simulink model "Y_Model_2_Loads"  (R2018b)
settings: Solver=VariableStepAuto  StartTime=0.0  StopTime=sim_t  RelTol=1e-3
values from neighbouring files (symbols this model uses):
  dt = 5e-5    (= 5e-05)    [Y_multi_sim_loads.m]
  L = ones(num_sims, num_loads) * L_max    [Y_multi_sim_loads.m]
  P = rand(num_sims, num_loads) * (P_max - P_min) + P_min    [Y_multi_sim_loads.m]
  R = ones(num_sims, num_loads) * R_max    [Y_multi_sim_loads.m]
libraries: powerlib x65, powerlib_meascontrol x13
settings Model: Creator=mitchell  LastModifiedBy=mitchell

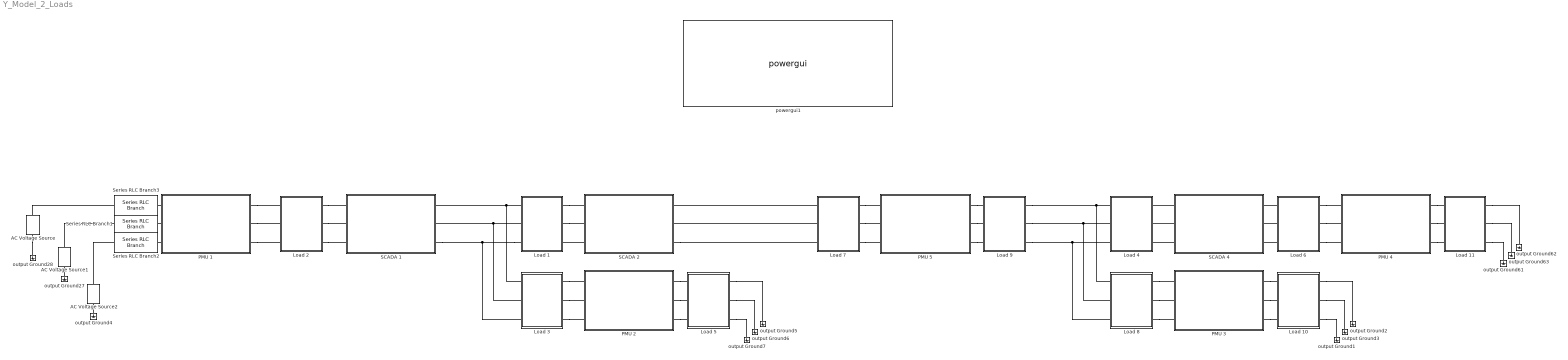
== system Y_Model_2_Loads ==
  AC Voltage Source : powerlib/Electrical Sources/AC Voltage Source  Amplitude=240  Phase=0  Frequency=50  SampleTime=0  Measurements=None  BusType=swing  Pref=10e3  Qref=0  Qmin=-inf  Qmax=+inf
  AC Voltage Source1 : powerlib/Electrical Sources/AC Voltage Source  Amplitude=240  Phase=-120  Frequency=50  SampleTime=0  Measurements=None  BusType=swing  Pref=10e3  Qref=0  Qmin=-inf  Qmax=+inf
  AC Voltage Source2 : powerlib/Electrical Sources/AC Voltage Source  Amplitude=240  Phase=-240  Frequency=50  SampleTime=0  Measurements=None  BusType=swing  Pref=10e3  Qref=0  Qmin=-inf  Qmax=+inf
  Load 1 : Subsystem
  Load 10 : Subsystem
  Load 11 : Subsystem
  Load 2 : Subsystem
  Load 3 : Subsystem
  Load 4 : Subsystem
  Load 5 : Subsystem
  Load 6 : Subsystem
  Load 7 : Subsystem
  Load 8 : Subsystem
  Load 9 : Subsystem
  PMU 1 : Subsystem
  PMU 2 : Subsystem
  PMU 3 : Subsystem
  PMU 4 : Subsystem
  PMU 5 : Subsystem
  SCADA 1 : Subsystem
  SCADA 2 : Subsystem
  SCADA 4 : Subsystem
  Series RLC Branch1 : powerlib/Elements/Series RLC Branch  LConnTagsString=__new0  RConnTagsString=__new0  BranchType=R  Resistance=1  Inductance=L(4)  SetiL0=off  InitialCurrent=0  Capacitance=0  Setx0=off  InitialVoltage=0  Measurements=None
  Series RLC Branch2 : powerlib/Elements/Series RLC Branch  LConnTagsString=__new0  RConnTagsString=__new0  BranchType=R  Resistance=1  Inductance=L(4)  SetiL0=off  InitialCurrent=0  Capacitance=0  Setx0=off  InitialVoltage=0  Measurements=None
  Series RLC Branch3 : powerlib/Elements/Series RLC Branch  LConnTagsString=__new0  RConnTagsString=__new0  BranchType=R  Resistance=1  Inductance=L(4)  SetiL0=off  InitialCurrent=0  Capacitance=0  Setx0=off  InitialVoltage=0  Measurements=None
  output Ground{1..7,27..28,61..63} (12 alike) : powerlib/Elements/Ground  LConnTagsString=a
      settings: SourceProductName=Simscape Electrical
  powergui1 : powerlib/powergui  Priority=1  SimulationMode=Discrete  SampleTime=dt  frequency=60  Iterations=500  frequencyindice=50  Pbase=100e6  ErrMax=0.0001  UnitsV=kV  UnitsW=MW  buscounter=1  FunctionMessages=off  echomessages=off  EnableUseOfTLC=off  CurrentSourceSwitches=off  DisableSnubberDevices=off  DisableRonSwitches=off  DisableVfSwitches=off  DisplayEquations=off  SolverType=Tustin/Backward Euler (TBE)  Interpol=off  ExternalGateDelay=off  methode=off  Ts=100  x0status=blocks  SPID=on  SwTol=0  HookPort=off  RestoreLinks=warning  ResistiveCurrentMeasurement=off  Frange=[0:2:500]  Ylog=off  Xlog=on  ShowGrid=off  save=off  variable=ZData  structure=0  ZoomFFT=off  StartTime=0.0  cycles=1  DisplayStyle=1  fundamental=60  FreqAxis=off  MaxFrequency=1000  frequencyindicesteady=1  RmsSteady=1  display=off
  connections:
  output Ground4/LConn1 -- AC Voltage Source2/LConn1
  output Ground27/LConn1 -- AC Voltage Source1/LConn1
  AC Voltage Source/LConn1 -- output Ground28/LConn1
  Series RLC Branch1/RConn1 -- PMU 1/LConn2
  Series RLC Branch2/RConn1 -- PMU 1/LConn3
  Load 3/LConn2 -- SCADA 1/RConn2 -- Load 1/LConn2
  Load 1/RConn1 -- SCADA 2/LConn1
  SCADA 2/LConn3 -- Load 1/RConn3
  AC Voltage Source2/RConn1 -- Series RLC Branch2/LConn1
  Series RLC Branch1/LConn1 -- AC Voltage Source1/RConn1
  Series RLC Branch3/LConn1 -- AC Voltage Source/RConn1
  PMU 1/LConn1 -- Series RLC Branch3/RConn1
  Load 1/LConn1 -- SCADA 1/RConn1 -- Load 3/LConn1
  PMU 1/RConn3 -- Load 2/LConn3
  PMU 1/RConn2 -- Load 2/LConn2
  PMU 1/RConn1 -- Load 2/LConn1
  Load 1/LConn3 -- SCADA 1/RConn3 -- Load 3/LConn3
  Load 2/RConn1 -- SCADA 1/LConn1
  Load 2/RConn2 -- SCADA 1/LConn2
  Load 2/RConn3 -- SCADA 1/LConn3
  Load 3/RConn1 -- PMU 2/LConn1
  Load 3/RConn2 -- PMU 2/LConn2
  Load 3/RConn3 -- PMU 2/LConn3
  PMU 2/RConn3 -- Load 5/LConn3
  PMU 2/RConn2 -- Load 5/LConn2
  PMU 2/RConn1 -- Load 5/LConn1
  Load 7/LConn2 -- SCADA 2/RConn2
  Load 7/LConn1 -- SCADA 2/RConn1
  SCADA 2/RConn3 -- Load 7/LConn3
  Load 7/RConn3 -- PMU 5/LConn3
  Load 7/RConn1 -- PMU 5/LConn1
  PMU 5/RConn2 -- Load 9/LConn2
  PMU 5/RConn1 -- Load 9/LConn1
  Load 7/RConn2 -- PMU 5/LConn2
  PMU 5/RConn3 -- Load 9/LConn3
  Load 1/RConn2 -- SCADA 2/LConn2
  Load 5/RConn2 -- output Ground6/LConn1
  Load 5/RConn1 -- output Ground5/LConn1
  Load 5/RConn3 -- output Ground7/LConn1
  Load 8/LConn2 -- Load 9/RConn2 -- Load 4/LConn2
  Load 4/LConn3 -- Load 9/RConn3 -- Load 8/LConn3
  Load 8/LConn1 -- Load 9/RConn1 -- Load 4/LConn1
  SCADA 4/LConn1 -- Load 4/RConn1
  Load 10/RConn3 -- output Ground1/LConn1
  Load 10/RConn2 -- output Ground3/LConn1
  SCADA 4/LConn3 -- Load 4/RConn3
  Load 10/RConn1 -- output Ground2/LConn1
  PMU 3/RConn2 -- Load 10/LConn2
  PMU 3/RConn3 -- Load 10/LConn3
  SCADA 4/LConn2 -- Load 4/RConn2
  Load 8/RConn1 -- PMU 3/LConn1
  PMU 3/RConn1 -- Load 10/LConn1
  Load 8/RConn2 -- PMU 3/LConn2
  Load 8/RConn3 -- PMU 3/LConn3
  Load 11/RConn2 -- output Ground63/LConn1
  Load 6/RConn1 -- PMU 4/LConn1
  PMU 4/RConn2 -- Load 11/LConn2
  Load 11/RConn3 -- output Ground61/LConn1
  PMU 4/RConn1 -- Load 11/LConn1
  Load 11/RConn1 -- output Ground62/LConn1
  PMU 4/RConn3 -- Load 11/LConn3
  Load 6/RConn2 -- PMU 4/LConn2
  Load 6/RConn3 -- PMU 4/LConn3
  Load 6/LConn1 -- SCADA 4/RConn1
  Load 6/LConn2 -- SCADA 4/RConn2
  Load 6/LConn3 -- SCADA 4/RConn3

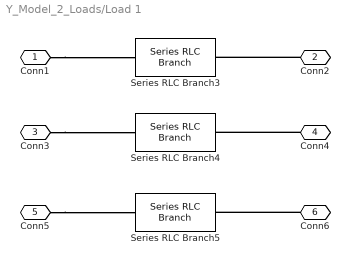
== system Y_Model_2_Loads/Load 1 ==
  Series RLC Branch3 : powerlib/Elements/Series RLC Branch  LConnTagsString=__new0  RConnTagsString=__new0  BranchType=RL  Resistance=R(1)  Inductance=L(1)  SetiL0=off  InitialCurrent=0  Capacitance=0  Setx0=off  InitialVoltage=0  Measurements=None
  Series RLC Branch4 : powerlib/Elements/Series RLC Branch  LConnTagsString=__new0  RConnTagsString=__new0  BranchType=RL  Resistance=R(1)  Inductance=L(1)  SetiL0=off  InitialCurrent=0  Capacitance=0  Setx0=off  InitialVoltage=0  Measurements=None
  Series RLC Branch5 : powerlib/Elements/Series RLC Branch  LConnTagsString=__new0  RConnTagsString=__new0  BranchType=RL  Resistance=R(1)  Inductance=L(1)  SetiL0=off  InitialCurrent=0  Capacitance=0  Setx0=off  InitialVoltage=0  Measurements=None
  Conn1 : PMIOPort  Side=Left
  Conn2 : PMIOPort  Port=2  Side=Right
  Conn3 : PMIOPort  Port=3  Side=Left
  Conn4 : PMIOPort  Port=4  Side=Right
  Conn5 : PMIOPort  Port=5  Side=Left
  Conn6 : PMIOPort  Port=6  Side=Right
  connections:
  Conn5/RConn1 -- Series RLC Branch5/LConn1
  Conn4/RConn1 -- Series RLC Branch4/RConn1
  Conn2/RConn1 -- Series RLC Branch3/RConn1
  Conn3/RConn1 -- Series RLC Branch4/LConn1
  Conn6/RConn1 -- Series RLC Branch5/RConn1
  Conn1/RConn1 -- Series RLC Branch3/LConn1

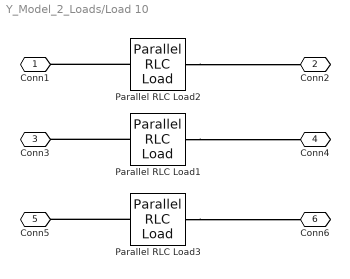
== system Y_Model_2_Loads/Load 10 ==
  Parallel RLC Load1 : powerlib/Elements/Parallel RLC Load  LConnTagsString=a  RConnTagsString=__new0  NominalVoltage=240  NominalFrequency=60  ActivePower=P(10)  InductivePower=P(10)/10  CapacitivePower=0  Setx0=off  InitialVoltage=0  SetiL0=off  InitialCurrent=0  Measurements=None  LoadType=constant Z
      settings: AttributesFormatString=\n  SourceProductName=Simscape Power Systems  SourceProductBaseCode=PS
  Parallel RLC Load2 : powerlib/Elements/Parallel RLC Load  LConnTagsString=a  RConnTagsString=__new0  NominalVoltage=240  NominalFrequency=60  ActivePower=P(10)  InductivePower=P(10)/10  CapacitivePower=0  Setx0=off  InitialVoltage=0  SetiL0=off  InitialCurrent=0  Measurements=None  LoadType=constant Z
      settings: AttributesFormatString=\n  SourceProductName=Simscape Power Systems  SourceProductBaseCode=PS
  Parallel RLC Load3 : powerlib/Elements/Parallel RLC Load  LConnTagsString=a  RConnTagsString=__new0  NominalVoltage=240  NominalFrequency=60  ActivePower=P(10)  InductivePower=P(10)/10  CapacitivePower=0  Setx0=off  InitialVoltage=0  SetiL0=off  InitialCurrent=0  Measurements=None  LoadType=constant Z
      settings: AttributesFormatString=\n  SourceProductName=Simscape Power Systems  SourceProductBaseCode=PS
  Conn1 : PMIOPort  Side=Left
  Conn2 : PMIOPort  Port=2  Side=Right
  Conn3 : PMIOPort  Port=3  Side=Left
  Conn4 : PMIOPort  Port=4  Side=Right
  Conn5 : PMIOPort  Port=5  Side=Left
  Conn6 : PMIOPort  Port=6  Side=Right
  connections:
  Parallel RLC Load3/LConn1 -- Conn5/RConn1
  Parallel RLC Load1/LConn1 -- Conn3/RConn1
  Parallel RLC Load2/LConn1 -- Conn1/RConn1
  Parallel RLC Load2/RConn1 -- Conn2/RConn1
  Parallel RLC Load1/RConn1 -- Conn4/RConn1
  Parallel RLC Load3/RConn1 -- Conn6/RConn1

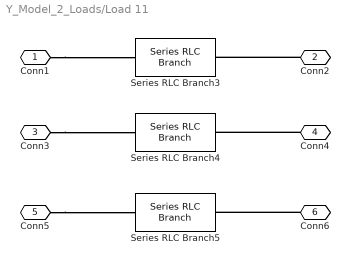
== system Y_Model_2_Loads/Load 11 ==
  Series RLC Branch3 : powerlib/Elements/Series RLC Branch  LConnTagsString=__new0  RConnTagsString=__new0  BranchType=RL  Resistance=R(4)  Inductance=L(4)  SetiL0=off  InitialCurrent=0  Capacitance=0  Setx0=off  InitialVoltage=0  Measurements=None
  Series RLC Branch4 : powerlib/Elements/Series RLC Branch  LConnTagsString=__new0  RConnTagsString=__new0  BranchType=RL  Resistance=R(4)  Inductance=L(4)  SetiL0=off  InitialCurrent=0  Capacitance=0  Setx0=off  InitialVoltage=0  Measurements=None
  Series RLC Branch5 : powerlib/Elements/Series RLC Branch  LConnTagsString=__new0  RConnTagsString=__new0  BranchType=RL  Resistance=R(4)  Inductance=L(4)  SetiL0=off  InitialCurrent=0  Capacitance=0  Setx0=off  InitialVoltage=0  Measurements=None
  Conn1 : PMIOPort  Side=Left
  Conn2 : PMIOPort  Port=2  Side=Right
  Conn3 : PMIOPort  Port=3  Side=Left
  Conn4 : PMIOPort  Port=4  Side=Right
  Conn5 : PMIOPort  Port=5  Side=Left
  Conn6 : PMIOPort  Port=6  Side=Right
  connections:
  Conn5/RConn1 -- Series RLC Branch5/LConn1
  Conn4/RConn1 -- Series RLC Branch4/RConn1
  Conn2/RConn1 -- Series RLC Branch3/RConn1
  Conn3/RConn1 -- Series RLC Branch4/LConn1
  Conn6/RConn1 -- Series RLC Branch5/RConn1
  Conn1/RConn1 -- Series RLC Branch3/LConn1

== system Y_Model_2_Loads/Load 2 ==
  Series RLC Branch3 : powerlib/Elements/Series RLC Branch  LConnTagsString=__new0  RConnTagsString=__new0  BranchType=RL  Resistance=R(2)  Inductance=L(2)  SetiL0=off  InitialCurrent=0  Capacitance=0  Setx0=off  InitialVoltage=0  Measurements=None
  Series RLC Branch4 : powerlib/Elements/Series RLC Branch  LConnTagsString=__new0  RConnTagsString=__new0  BranchType=RL  Resistance=R(2)  Inductance=L(2)  SetiL0=off  InitialCurrent=0  Capacitance=0  Setx0=off  InitialVoltage=0  Measurements=None
  Series RLC Branch5 : powerlib/Elements/Series RLC Branch  LConnTagsString=__new0  RConnTagsString=__new0  BranchType=RL  Resistance=R(2)  Inductance=L(2)  SetiL0=off  InitialCurrent=0  Capacitance=0  Setx0=off  InitialVoltage=0  Measurements=None
  Conn1 : PMIOPort  Side=Left
  Conn2 : PMIOPort  Port=2  Side=Right
  Conn3 : PMIOPort  Port=3  Side=Left
  Conn4 : PMIOPort  Port=4  Side=Right
  Conn5 : PMIOPort  Port=5  Side=Left
  Conn6 : PMIOPort  Port=6  Side=Right
  connections:
  Conn5/RConn1 -- Series RLC Branch5/LConn1
  Conn4/RConn1 -- Series RLC Branch4/RConn1
  Conn2/RConn1 -- Series RLC Branch3/RConn1
  Conn3/RConn1 -- Series RLC Branch4/LConn1
  Conn6/RConn1 -- Series RLC Branch5/RConn1
  Conn1/RConn1 -- Series RLC Branch3/LConn1

== system Y_Model_2_Loads/Load 3 ==
  Series RLC Branch3 : powerlib/Elements/Series RLC Branch  LConnTagsString=__new0  RConnTagsString=__new0  BranchType=RL  Resistance=R(3)  Inductance=L(3)  SetiL0=off  InitialCurrent=0  Capacitance=0  Setx0=off  InitialVoltage=0  Measurements=None
  Series RLC Branch4 : powerlib/Elements/Series RLC Branch  LConnTagsString=__new0  RConnTagsString=__new0  BranchType=RL  Resistance=R(3)  Inductance=L(3)  SetiL0=off  InitialCurrent=0  Capacitance=0  Setx0=off  InitialVoltage=0  Measurements=None
  Series RLC Branch5 : powerlib/Elements/Series RLC Branch  LConnTagsString=__new0  RConnTagsString=__new0  BranchType=RL  Resistance=R(3)  Inductance=L(3)  SetiL0=off  InitialCurrent=0  Capacitance=0  Setx0=off  InitialVoltage=0  Measurements=None
  Conn1 : PMIOPort  Side=Left
  Conn2 : PMIOPort  Port=2  Side=Right
  Conn3 : PMIOPort  Port=3  Side=Left
  Conn4 : PMIOPort  Port=4  Side=Right
  Conn5 : PMIOPort  Port=5  Side=Left
  Conn6 : PMIOPort  Port=6  Side=Right
  connections:
  Conn5/RConn1 -- Series RLC Branch5/LConn1
  Conn4/RConn1 -- Series RLC Branch4/RConn1
  Conn2/RConn1 -- Series RLC Branch3/RConn1
  Conn3/RConn1 -- Series RLC Branch4/LConn1
  Conn6/RConn1 -- Series RLC Branch5/RConn1
  Conn1/RConn1 -- Series RLC Branch3/LConn1

== system Y_Model_2_Loads/Load 4 ==
  Series RLC Branch3 : powerlib/Elements/Series RLC Branch  LConnTagsString=__new0  RConnTagsString=__new0  BranchType=RL  Resistance=R(1)  Inductance=L(1)  SetiL0=off  InitialCurrent=0  Capacitance=0  Setx0=off  InitialVoltage=0  Measurements=None
  Series RLC Branch4 : powerlib/Elements/Series RLC Branch  LConnTagsString=__new0  RConnTagsString=__new0  BranchType=RL  Resistance=R(1)  Inductance=L(1)  SetiL0=off  InitialCurrent=0  Capacitance=0  Setx0=off  InitialVoltage=0  Measurements=None
  Series RLC Branch5 : powerlib/Elements/Series RLC Branch  LConnTagsString=__new0  RConnTagsString=__new0  BranchType=RL  Resistance=R(1)  Inductance=L(1)  SetiL0=off  InitialCurrent=0  Capacitance=0  Setx0=off  InitialVoltage=0  Measurements=None
  Conn1 : PMIOPort  Side=Left
  Conn2 : PMIOPort  Port=2  Side=Right
  Conn3 : PMIOPort  Port=3  Side=Left
  Conn4 : PMIOPort  Port=4  Side=Right
  Conn5 : PMIOPort  Port=5  Side=Left
  Conn6 : PMIOPort  Port=6  Side=Right
  connections:
  Conn5/RConn1 -- Series RLC Branch5/LConn1
  Conn4/RConn1 -- Series RLC Branch4/RConn1
  Conn2/RConn1 -- Series RLC Branch3/RConn1
  Conn3/RConn1 -- Series RLC Branch4/LConn1
  Conn6/RConn1 -- Series RLC Branch5/RConn1
  Conn1/RConn1 -- Series RLC Branch3/LConn1

== system Y_Model_2_Loads/Load 5 ==
  Parallel RLC Load1 : powerlib/Elements/Parallel RLC Load  LConnTagsString=a  RConnTagsString=__new0  NominalVoltage=240  NominalFrequency=60  ActivePower=P(5)  InductivePower=P(5)/10  CapacitivePower=0  Setx0=off  InitialVoltage=0  SetiL0=off  InitialCurrent=0  Measurements=None  LoadType=constant Z
      settings: AttributesFormatString=\n  SourceProductName=Simscape Power Systems  SourceProductBaseCode=PS
  Parallel RLC Load2 : powerlib/Elements/Parallel RLC Load  LConnTagsString=a  RConnTagsString=__new0  NominalVoltage=240  NominalFrequency=60  ActivePower=P(5)  InductivePower=P(5)/10  CapacitivePower=0  Setx0=off  InitialVoltage=0  SetiL0=off  InitialCurrent=0  Measurements=None  LoadType=constant Z
      settings: AttributesFormatString=\n  SourceProductName=Simscape Power Systems  SourceProductBaseCode=PS
  Parallel RLC Load3 : powerlib/Elements/Parallel RLC Load  LConnTagsString=a  RConnTagsString=__new0  NominalVoltage=240  NominalFrequency=60  ActivePower=P(5)  InductivePower=P(5)/10  CapacitivePower=0  Setx0=off  InitialVoltage=0  SetiL0=off  InitialCurrent=0  Measurements=None  LoadType=constant Z
      settings: AttributesFormatString=\n  SourceProductName=Simscape Power Systems  SourceProductBaseCode=PS
  Conn1 : PMIOPort  Side=Left
  Conn2 : PMIOPort  Port=2  Side=Right
  Conn3 : PMIOPort  Port=3  Side=Left
  Conn4 : PMIOPort  Port=4  Side=Right
  Conn5 : PMIOPort  Port=5  Side=Left
  Conn6 : PMIOPort  Port=6  Side=Right
  connections:
  Parallel RLC Load2/LConn1 -- Conn5/RConn1
  Conn4/RConn1 -- Parallel RLC Load1/RConn1
  Parallel RLC Load3/RConn1 -- Conn2/RConn1
  Parallel RLC Load1/LConn1 -- Conn3/RConn1
  Conn6/RConn1 -- Parallel RLC Load2/RConn1
  Parallel RLC Load3/LConn1 -- Conn1/RConn1

== system Y_Model_2_Loads/Load 6 ==
  Series RLC Branch3 : powerlib/Elements/Series RLC Branch  LConnTagsString=__new0  RConnTagsString=__new0  BranchType=RL  Resistance=R(3)  Inductance=L(3)  SetiL0=off  InitialCurrent=0  Capacitance=0  Setx0=off  InitialVoltage=0  Measurements=None
  Series RLC Branch4 : powerlib/Elements/Series RLC Branch  LConnTagsString=__new0  RConnTagsString=__new0  BranchType=RL  Resistance=R(3)  Inductance=L(3)  SetiL0=off  InitialCurrent=0  Capacitance=0  Setx0=off  InitialVoltage=0  Measurements=None
  Series RLC Branch5 : powerlib/Elements/Series RLC Branch  LConnTagsString=__new0  RConnTagsString=__new0  BranchType=RL  Resistance=R(3)  Inductance=L(3)  SetiL0=off  InitialCurrent=0  Capacitance=0  Setx0=off  InitialVoltage=0  Measurements=None
  Conn1 : PMIOPort  Side=Left
  Conn2 : PMIOPort  Port=2  Side=Right
  Conn3 : PMIOPort  Port=3  Side=Left
  Conn4 : PMIOPort  Port=4  Side=Right
  Conn5 : PMIOPort  Port=5  Side=Left
  Conn6 : PMIOPort  Port=6  Side=Right
  connections:
  Conn5/RConn1 -- Series RLC Branch5/LConn1
  Conn4/RConn1 -- Series RLC Branch4/RConn1
  Conn2/RConn1 -- Series RLC Branch3/RConn1
  Conn3/RConn1 -- Series RLC Branch4/LConn1
  Conn6/RConn1 -- Series RLC Branch5/RConn1
  Conn1/RConn1 -- Series RLC Branch3/LConn1

== system Y_Model_2_Loads/Load 7 ==
  Series RLC Branch3 : powerlib/Elements/Series RLC Branch  LConnTagsString=__new0  RConnTagsString=__new0  BranchType=RL  Resistance=R(3)  Inductance=L(3)  SetiL0=off  InitialCurrent=0  Capacitance=0  Setx0=off  InitialVoltage=0  Measurements=None
  Series RLC Branch4 : powerlib/Elements/Series RLC Branch  LConnTagsString=__new0  RConnTagsString=__new0  BranchType=RL  Resistance=R(3)  Inductance=L(3)  SetiL0=off  InitialCurrent=0  Capacitance=0  Setx0=off  InitialVoltage=0  Measurements=None
  Series RLC Branch5 : powerlib/Elements/Series RLC Branch  LConnTagsString=__new0  RConnTagsString=__new0  BranchType=RL  Resistance=R(3)  Inductance=L(3)  SetiL0=off  InitialCurrent=0  Capacitance=0  Setx0=off  InitialVoltage=0  Measurements=None
  Conn1 : PMIOPort  Side=Left
  Conn2 : PMIOPort  Port=2  Side=Right
  Conn3 : PMIOPort  Port=3  Side=Left
  Conn4 : PMIOPort  Port=4  Side=Right
  Conn5 : PMIOPort  Port=5  Side=Left
  Conn6 : PMIOPort  Port=6  Side=Right
  connections:
  Conn5/RConn1 -- Series RLC Branch5/LConn1
  Conn4/RConn1 -- Series RLC Branch4/RConn1
  Conn2/RConn1 -- Series RLC Branch3/RConn1
  Conn3/RConn1 -- Series RLC Branch4/LConn1
  Conn6/RConn1 -- Series RLC Branch5/RConn1
  Conn1/RConn1 -- Series RLC Branch3/LConn1

== system Y_Model_2_Loads/Load 8 ==
  Series RLC Branch3 : powerlib/Elements/Series RLC Branch  LConnTagsString=__new0  RConnTagsString=__new0  BranchType=RL  Resistance=R(3)  Inductance=L(3)  SetiL0=off  InitialCurrent=0  Capacitance=0  Setx0=off  InitialVoltage=0  Measurements=None
  Series RLC Branch4 : powerlib/Elements/Series RLC Branch  LConnTagsString=__new0  RConnTagsString=__new0  BranchType=RL  Resistance=R(3)  Inductance=L(3)  SetiL0=off  InitialCurrent=0  Capacitance=0  Setx0=off  InitialVoltage=0  Measurements=None
  Series RLC Branch5 : powerlib/Elements/Series RLC Branch  LConnTagsString=__new0  RConnTagsString=__new0  BranchType=RL  Resistance=R(3)  Inductance=L(3)  SetiL0=off  InitialCurrent=0  Capacitance=0  Setx0=off  InitialVoltage=0  Measurements=None
  Conn1 : PMIOPort  Side=Left
  Conn2 : PMIOPort  Port=2  Side=Right
  Conn3 : PMIOPort  Port=3  Side=Left
  Conn4 : PMIOPort  Port=4  Side=Right
  Conn5 : PMIOPort  Port=5  Side=Left
  Conn6 : PMIOPort  Port=6  Side=Right
  connections:
  Conn5/RConn1 -- Series RLC Branch5/LConn1
  Conn4/RConn1 -- Series RLC Branch4/RConn1
  Conn2/RConn1 -- Series RLC Branch3/RConn1
  Conn3/RConn1 -- Series RLC Branch4/LConn1
  Conn6/RConn1 -- Series RLC Branch5/RConn1
  Conn1/RConn1 -- Series RLC Branch3/LConn1

== system Y_Model_2_Loads/Load 9 ==
  Series RLC Branch3 : powerlib/Elements/Series RLC Branch  LConnTagsString=__new0  RConnTagsString=__new0  BranchType=RL  Resistance=R(4)  Inductance=L(4)  SetiL0=off  InitialCurrent=0  Capacitance=0  Setx0=off  InitialVoltage=0  Measurements=None
  Series RLC Branch4 : powerlib/Elements/Series RLC Branch  LConnTagsString=__new0  RConnTagsString=__new0  BranchType=RL  Resistance=R(4)  Inductance=L(4)  SetiL0=off  InitialCurrent=0  Capacitance=0  Setx0=off  InitialVoltage=0  Measurements=None
  Series RLC Branch5 : powerlib/Elements/Series RLC Branch  LConnTagsString=__new0  RConnTagsString=__new0  BranchType=RL  Resistance=R(4)  Inductance=L(4)  SetiL0=off  InitialCurrent=0  Capacitance=0  Setx0=off  InitialVoltage=0  Measurements=None
  Conn1 : PMIOPort  Side=Left
  Conn2 : PMIOPort  Port=2  Side=Right
  Conn3 : PMIOPort  Port=3  Side=Left
  Conn4 : PMIOPort  Port=4  Side=Right
  Conn5 : PMIOPort  Port=5  Side=Left
  Conn6 : PMIOPort  Port=6  Side=Right
  connections:
  Conn5/RConn1 -- Series RLC Branch5/LConn1
  Conn4/RConn1 -- Series RLC Branch4/RConn1
  Conn2/RConn1 -- Series RLC Branch3/RConn1
  Conn3/RConn1 -- Series RLC Branch4/LConn1
  Conn6/RConn1 -- Series RLC Branch5/RConn1
  Conn1/RConn1 -- Series RLC Branch3/LConn1

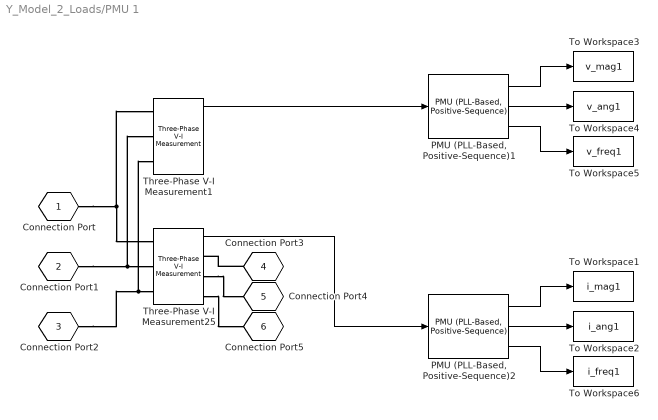
== system Y_Model_2_Loads/PMU 1 ==
  "PMU (PLL-Based, Positive-Sequence)1" : powerlib_meascontrol/Measurements/PMU (PLL-Based, Positive-Sequence)  nominalFrequency=50  samplingRate=64  reportingFactor=64
      settings: SourceProductName=Simscape Electrical  SourceProductBaseCode=PS
  "PMU (PLL-Based, Positive-Sequence)2" : powerlib_meascontrol/Measurements/PMU (PLL-Based, Positive-Sequence)  nominalFrequency=50  samplingRate=64  reportingFactor=64
      settings: SourceProductName=Simscape Electrical  SourceProductBaseCode=PS
  Three-Phase V-I Measurement1 : powerlib/Measurements/Three-Phase V-I Measurement  VoltageMeasurement=phase-to-ground  SetLabelV=off  LabelV=Vabc  Vpu=off  VpuLL=off  CurrentMeasurement=no  SetLabelI=off  LabelI=Iabc  Ipu=off  Pbase=100e6  Vbase=500e3  OutputType=Complex  PhasorSimulation=off  PSBequivalent=0
      settings: SourceProductName=Simscape Electrical
  Three-Phase V-I Measurement25 : powerlib/Measurements/Three-Phase V-I Measurement  VoltageMeasurement=no  SetLabelV=off  LabelV=Vabc  Vpu=off  VpuLL=off  CurrentMeasurement=yes  SetLabelI=off  LabelI=Iabc  Ipu=off  Pbase=100e6  Vbase=500e3  OutputType=Complex  PhasorSimulation=off  PSBequivalent=0
      settings: SourceProductName=Simscape Electrical
  To Workspace1 : ToWorkspace  VariableName=i_mag1  SampleTime=-1
  To Workspace2 : ToWorkspace  VariableName=i_ang1  SampleTime=-1
  To Workspace3 : ToWorkspace  VariableName=v_mag1  SampleTime=-1
  To Workspace4 : ToWorkspace  VariableName=v_ang1  SampleTime=-1
  To Workspace5 : ToWorkspace  VariableName=v_freq1  SampleTime=-1
  To Workspace6 : ToWorkspace  VariableName=i_freq1  SampleTime=-1
  Connection Port : PMIOPort  Tag=PMCPort  Side=Left
  Connection Port1 : PMIOPort  Tag=PMCPort  Port=2  Side=Left
  Connection Port2 : PMIOPort  Tag=PMCPort  Port=3  Side=Left
  Connection Port3 : PMIOPort  Tag=PMCPort  Port=4  Side=Right
  Connection Port4 : PMIOPort  Tag=PMCPort  Port=5  Side=Right
  Connection Port5 : PMIOPort  Tag=PMCPort  Port=6  Side=Right
  wires:
  "PMU (PLL-Based, Positive-Sequence)1"/3 -> To Workspace5/1
  "PMU (PLL-Based, Positive-Sequence)1"/2 -> To Workspace4/1
  "PMU (PLL-Based, Positive-Sequence)1"/1 -> To Workspace3/1
  "PMU (PLL-Based, Positive-Sequence)2"/3 -> To Workspace6/1
  "PMU (PLL-Based, Positive-Sequence)2"/1 -> To Workspace1/1
  "PMU (PLL-Based, Positive-Sequence)2"/2 -> To Workspace2/1
  Three-Phase V-I Measurement25/1 -> "PMU (PLL-Based, Positive-Sequence)2"/1
  Three-Phase V-I Measurement1/1 -> "PMU (PLL-Based, Positive-Sequence)1"/1
  connections:
  Connection Port/RConn1 -- Three-Phase V-I Measurement1/LConn1 -- Three-Phase V-I Measurement25/LConn1
  Connection Port1/RConn1 -- Three-Phase V-I Measurement25/LConn2 -- Three-Phase V-I Measurement1/LConn2
  Connection Port2/RConn1 -- Three-Phase V-I Measurement1/LConn3 -- Three-Phase V-I Measurement25/LConn3
  Connection Port3/RConn1 -- Three-Phase V-I Measurement25/RConn1
  Three-Phase V-I Measurement25/RConn2 -- Connection Port4/RConn1
  Three-Phase V-I Measurement25/RConn3 -- Connection Port5/RConn1

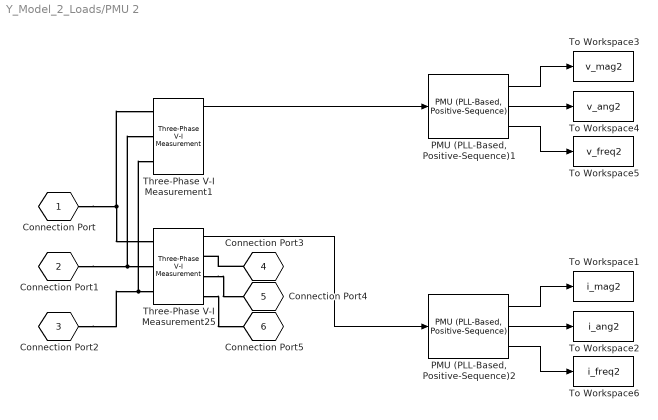
== system Y_Model_2_Loads/PMU 2 ==
  "PMU (PLL-Based, Positive-Sequence)1" : powerlib_meascontrol/Measurements/PMU (PLL-Based, Positive-Sequence)  nominalFrequency=50  samplingRate=64  reportingFactor=64
      settings: SourceProductName=Simscape Electrical  SourceProductBaseCode=PS
  "PMU (PLL-Based, Positive-Sequence)2" : powerlib_meascontrol/Measurements/PMU (PLL-Based, Positive-Sequence)  nominalFrequency=50  samplingRate=64  reportingFactor=64
      settings: SourceProductName=Simscape Electrical  SourceProductBaseCode=PS
  Three-Phase V-I Measurement1 : powerlib/Measurements/Three-Phase V-I Measurement  VoltageMeasurement=phase-to-ground  SetLabelV=off  LabelV=Vabc  Vpu=off  VpuLL=off  CurrentMeasurement=no  SetLabelI=off  LabelI=Iabc  Ipu=off  Pbase=100e6  Vbase=500e3  OutputType=Complex  PhasorSimulation=off  PSBequivalent=0
      settings: SourceProductName=Simscape Electrical
  Three-Phase V-I Measurement25 : powerlib/Measurements/Three-Phase V-I Measurement  VoltageMeasurement=no  SetLabelV=off  LabelV=Vabc  Vpu=off  VpuLL=off  CurrentMeasurement=yes  SetLabelI=off  LabelI=Iabc  Ipu=off  Pbase=100e6  Vbase=500e3  OutputType=Complex  PhasorSimulation=off  PSBequivalent=0
      settings: SourceProductName=Simscape Electrical
  To Workspace1 : ToWorkspace  VariableName=i_mag2  SampleTime=-1
  To Workspace2 : ToWorkspace  VariableName=i_ang2  SampleTime=-1
  To Workspace3 : ToWorkspace  VariableName=v_mag2  SampleTime=-1
  To Workspace4 : ToWorkspace  VariableName=v_ang2  SampleTime=-1
  To Workspace5 : ToWorkspace  VariableName=v_freq2  SampleTime=-1
  To Workspace6 : ToWorkspace  VariableName=i_freq2  SampleTime=-1
  Connection Port : PMIOPort  Tag=PMCPort  Side=Left
  Connection Port1 : PMIOPort  Tag=PMCPort  Port=2  Side=Left
  Connection Port2 : PMIOPort  Tag=PMCPort  Port=3  Side=Left
  Connection Port3 : PMIOPort  Tag=PMCPort  Port=4  Side=Right
  Connection Port4 : PMIOPort  Tag=PMCPort  Port=5  Side=Right
  Connection Port5 : PMIOPort  Tag=PMCPort  Port=6  Side=Right
  wires:
  "PMU (PLL-Based, Positive-Sequence)1"/3 -> To Workspace5/1
  "PMU (PLL-Based, Positive-Sequence)1"/2 -> To Workspace4/1
  "PMU (PLL-Based, Positive-Sequence)1"/1 -> To Workspace3/1
  "PMU (PLL-Based, Positive-Sequence)2"/3 -> To Workspace6/1
  "PMU (PLL-Based, Positive-Sequence)2"/1 -> To Workspace1/1
  "PMU (PLL-Based, Positive-Sequence)2"/2 -> To Workspace2/1
  Three-Phase V-I Measurement25/1 -> "PMU (PLL-Based, Positive-Sequence)2"/1
  Three-Phase V-I Measurement1/1 -> "PMU (PLL-Based, Positive-Sequence)1"/1
  connections:
  Three-Phase V-I Measurement25/LConn1 -- Connection Port/RConn1 -- Three-Phase V-I Measurement1/LConn1
  Connection Port1/RConn1 -- Three-Phase V-I Measurement1/LConn2 -- Three-Phase V-I Measurement25/LConn2
  Connection Port2/RConn1 -- Three-Phase V-I Measurement25/LConn3 -- Three-Phase V-I Measurement1/LConn3
  Connection Port3/RConn1 -- Three-Phase V-I Measurement25/RConn1
  Three-Phase V-I Measurement25/RConn2 -- Connection Port4/RConn1
  Three-Phase V-I Measurement25/RConn3 -- Connection Port5/RConn1

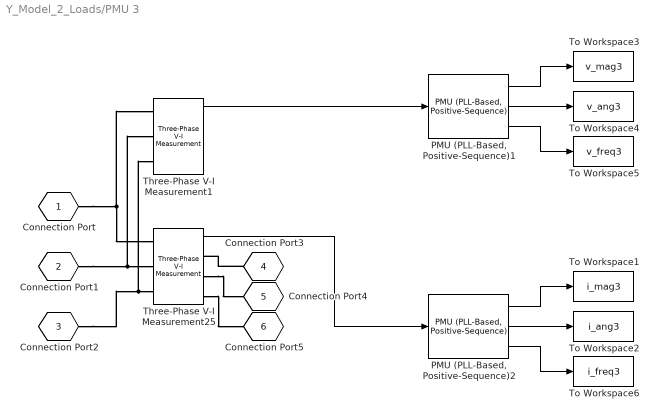
== system Y_Model_2_Loads/PMU 3 ==
  "PMU (PLL-Based, Positive-Sequence)1" : powerlib_meascontrol/Measurements/PMU (PLL-Based, Positive-Sequence)  nominalFrequency=50  samplingRate=64  reportingFactor=64
      settings: SourceProductName=Simscape Electrical  SourceProductBaseCode=PS
  "PMU (PLL-Based, Positive-Sequence)2" : powerlib_meascontrol/Measurements/PMU (PLL-Based, Positive-Sequence)  nominalFrequency=50  samplingRate=64  reportingFactor=64
      settings: SourceProductName=Simscape Electrical  SourceProductBaseCode=PS
  Three-Phase V-I Measurement1 : powerlib/Measurements/Three-Phase V-I Measurement  VoltageMeasurement=phase-to-ground  SetLabelV=off  LabelV=Vabc  Vpu=off  VpuLL=off  CurrentMeasurement=no  SetLabelI=off  LabelI=Iabc  Ipu=off  Pbase=100e6  Vbase=500e3  OutputType=Complex  PhasorSimulation=off  PSBequivalent=0
      settings: SourceProductName=Simscape Electrical
  Three-Phase V-I Measurement25 : powerlib/Measurements/Three-Phase V-I Measurement  VoltageMeasurement=no  SetLabelV=off  LabelV=Vabc  Vpu=off  VpuLL=off  CurrentMeasurement=yes  SetLabelI=off  LabelI=Iabc  Ipu=off  Pbase=100e6  Vbase=500e3  OutputType=Complex  PhasorSimulation=off  PSBequivalent=0
      settings: SourceProductName=Simscape Electrical
  To Workspace1 : ToWorkspace  VariableName=i_mag3  SampleTime=-1
  To Workspace2 : ToWorkspace  VariableName=i_ang3  SampleTime=-1
  To Workspace3 : ToWorkspace  VariableName=v_mag3  SampleTime=-1
  To Workspace4 : ToWorkspace  VariableName=v_ang3  SampleTime=-1
  To Workspace5 : ToWorkspace  VariableName=v_freq3  SampleTime=-1
  To Workspace6 : ToWorkspace  VariableName=i_freq3  SampleTime=-1
  Connection Port : PMIOPort  Tag=PMCPort  Side=Left
  Connection Port1 : PMIOPort  Tag=PMCPort  Port=2  Side=Left
  Connection Port2 : PMIOPort  Tag=PMCPort  Port=3  Side=Left
  Connection Port3 : PMIOPort  Tag=PMCPort  Port=4  Side=Right
  Connection Port4 : PMIOPort  Tag=PMCPort  Port=5  Side=Right
  Connection Port5 : PMIOPort  Tag=PMCPort  Port=6  Side=Right
  wires:
  "PMU (PLL-Based, Positive-Sequence)1"/3 -> To Workspace5/1
  "PMU (PLL-Based, Positive-Sequence)1"/2 -> To Workspace4/1
  "PMU (PLL-Based, Positive-Sequence)1"/1 -> To Workspace3/1
  "PMU (PLL-Based, Positive-Sequence)2"/3 -> To Workspace6/1
  "PMU (PLL-Based, Positive-Sequence)2"/1 -> To Workspace1/1
  "PMU (PLL-Based, Positive-Sequence)2"/2 -> To Workspace2/1
  Three-Phase V-I Measurement25/1 -> "PMU (PLL-Based, Positive-Sequence)2"/1
  Three-Phase V-I Measurement1/1 -> "PMU (PLL-Based, Positive-Sequence)1"/1
  connections:
  Three-Phase V-I Measurement25/LConn1 -- Connection Port/RConn1 -- Three-Phase V-I Measurement1/LConn1
  Connection Port1/RConn1 -- Three-Phase V-I Measurement1/LConn2 -- Three-Phase V-I Measurement25/LConn2
  Connection Port2/RConn1 -- Three-Phase V-I Measurement25/LConn3 -- Three-Phase V-I Measurement1/LConn3
  Connection Port3/RConn1 -- Three-Phase V-I Measurement25/RConn1
  Three-Phase V-I Measurement25/RConn2 -- Connection Port4/RConn1
  Three-Phase V-I Measurement25/RConn3 -- Connection Port5/RConn1

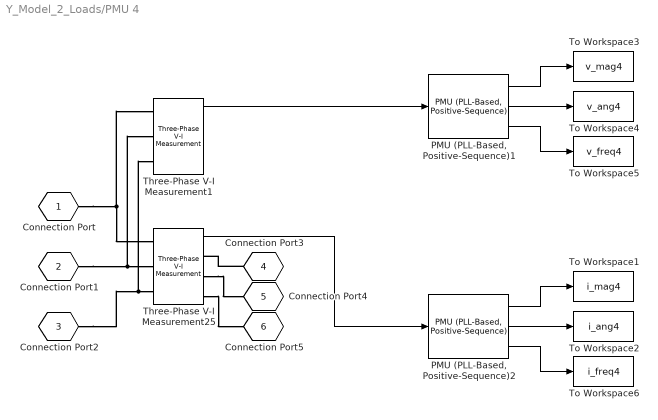
== system Y_Model_2_Loads/PMU 4 ==
  "PMU (PLL-Based, Positive-Sequence)1" : powerlib_meascontrol/Measurements/PMU (PLL-Based, Positive-Sequence)  nominalFrequency=50  samplingRate=64  reportingFactor=64
      settings: SourceProductName=Simscape Electrical  SourceProductBaseCode=PS
  "PMU (PLL-Based, Positive-Sequence)2" : powerlib_meascontrol/Measurements/PMU (PLL-Based, Positive-Sequence)  nominalFrequency=50  samplingRate=64  reportingFactor=64
      settings: SourceProductName=Simscape Electrical  SourceProductBaseCode=PS
  Three-Phase V-I Measurement1 : powerlib/Measurements/Three-Phase V-I Measurement  VoltageMeasurement=phase-to-ground  SetLabelV=off  LabelV=Vabc  Vpu=off  VpuLL=off  CurrentMeasurement=no  SetLabelI=off  LabelI=Iabc  Ipu=off  Pbase=100e6  Vbase=500e3  OutputType=Complex  PhasorSimulation=off  PSBequivalent=0
      settings: SourceProductName=Simscape Electrical
  Three-Phase V-I Measurement25 : powerlib/Measurements/Three-Phase V-I Measurement  VoltageMeasurement=no  SetLabelV=off  LabelV=Vabc  Vpu=off  VpuLL=off  CurrentMeasurement=yes  SetLabelI=off  LabelI=Iabc  Ipu=off  Pbase=100e6  Vbase=500e3  OutputType=Complex  PhasorSimulation=off  PSBequivalent=0
      settings: SourceProductName=Simscape Electrical
  To Workspace1 : ToWorkspace  VariableName=i_mag4  SampleTime=-1
  To Workspace2 : ToWorkspace  VariableName=i_ang4  SampleTime=-1
  To Workspace3 : ToWorkspace  VariableName=v_mag4  SampleTime=-1
  To Workspace4 : ToWorkspace  VariableName=v_ang4  SampleTime=-1
  To Workspace5 : ToWorkspace  VariableName=v_freq4  SampleTime=-1
  To Workspace6 : ToWorkspace  VariableName=i_freq4  SampleTime=-1
  Connection Port : PMIOPort  Tag=PMCPort  Side=Left
  Connection Port1 : PMIOPort  Tag=PMCPort  Port=2  Side=Left
  Connection Port2 : PMIOPort  Tag=PMCPort  Port=3  Side=Left
  Connection Port3 : PMIOPort  Tag=PMCPort  Port=4  Side=Right
  Connection Port4 : PMIOPort  Tag=PMCPort  Port=5  Side=Right
  Connection Port5 : PMIOPort  Tag=PMCPort  Port=6  Side=Right
  wires:
  "PMU (PLL-Based, Positive-Sequence)1"/3 -> To Workspace5/1
  "PMU (PLL-Based, Positive-Sequence)1"/2 -> To Workspace4/1
  "PMU (PLL-Based, Positive-Sequence)1"/1 -> To Workspace3/1
  "PMU (PLL-Based, Positive-Sequence)2"/3 -> To Workspace6/1
  "PMU (PLL-Based, Positive-Sequence)2"/1 -> To Workspace1/1
  "PMU (PLL-Based, Positive-Sequence)2"/2 -> To Workspace2/1
  Three-Phase V-I Measurement25/1 -> "PMU (PLL-Based, Positive-Sequence)2"/1
  Three-Phase V-I Measurement1/1 -> "PMU (PLL-Based, Positive-Sequence)1"/1
  connections:
  Three-Phase V-I Measurement25/LConn1 -- Connection Port/RConn1 -- Three-Phase V-I Measurement1/LConn1
  Connection Port1/RConn1 -- Three-Phase V-I Measurement1/LConn2 -- Three-Phase V-I Measurement25/LConn2
  Connection Port2/RConn1 -- Three-Phase V-I Measurement25/LConn3 -- Three-Phase V-I Measurement1/LConn3
  Connection Port3/RConn1 -- Three-Phase V-I Measurement25/RConn1
  Three-Phase V-I Measurement25/RConn2 -- Connection Port4/RConn1
  Three-Phase V-I Measurement25/RConn3 -- Connection Port5/RConn1

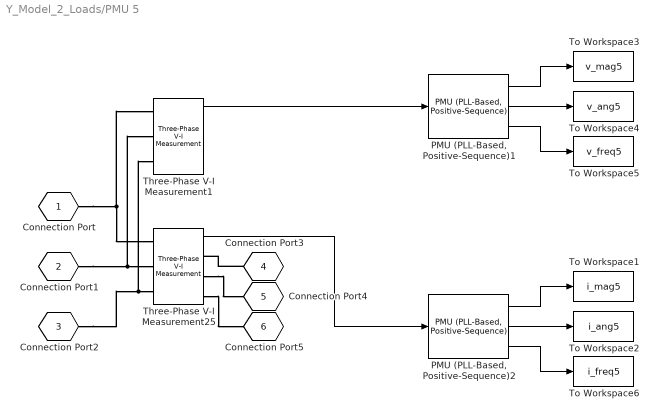
== system Y_Model_2_Loads/PMU 5 ==
  "PMU (PLL-Based, Positive-Sequence)1" : powerlib_meascontrol/Measurements/PMU (PLL-Based, Positive-Sequence)  nominalFrequency=50  samplingRate=64  reportingFactor=64
      settings: SourceProductName=Simscape Electrical  SourceProductBaseCode=PS
  "PMU (PLL-Based, Positive-Sequence)2" : powerlib_meascontrol/Measurements/PMU (PLL-Based, Positive-Sequence)  nominalFrequency=50  samplingRate=64  reportingFactor=64
      settings: SourceProductName=Simscape Electrical  SourceProductBaseCode=PS
  Three-Phase V-I Measurement1 : powerlib/Measurements/Three-Phase V-I Measurement  VoltageMeasurement=phase-to-ground  SetLabelV=off  LabelV=Vabc  Vpu=off  VpuLL=off  CurrentMeasurement=no  SetLabelI=off  LabelI=Iabc  Ipu=off  Pbase=100e6  Vbase=500e3  OutputType=Complex  PhasorSimulation=off  PSBequivalent=0
      settings: SourceProductName=Simscape Electrical
  Three-Phase V-I Measurement25 : powerlib/Measurements/Three-Phase V-I Measurement  VoltageMeasurement=no  SetLabelV=off  LabelV=Vabc  Vpu=off  VpuLL=off  CurrentMeasurement=yes  SetLabelI=off  LabelI=Iabc  Ipu=off  Pbase=100e6  Vbase=500e3  OutputType=Complex  PhasorSimulation=off  PSBequivalent=0
      settings: SourceProductName=Simscape Electrical
  To Workspace1 : ToWorkspace  VariableName=i_mag5  SampleTime=-1
  To Workspace2 : ToWorkspace  VariableName=i_ang5  SampleTime=-1
  To Workspace3 : ToWorkspace  VariableName=v_mag5  SampleTime=-1
  To Workspace4 : ToWorkspace  VariableName=v_ang5  SampleTime=-1
  To Workspace5 : ToWorkspace  VariableName=v_freq5  SampleTime=-1
  To Workspace6 : ToWorkspace  VariableName=i_freq5  SampleTime=-1
  Connection Port : PMIOPort  Tag=PMCPort  Side=Left
  Connection Port1 : PMIOPort  Tag=PMCPort  Port=2  Side=Left
  Connection Port2 : PMIOPort  Tag=PMCPort  Port=3  Side=Left
  Connection Port3 : PMIOPort  Tag=PMCPort  Port=4  Side=Right
  Connection Port4 : PMIOPort  Tag=PMCPort  Port=5  Side=Right
  Connection Port5 : PMIOPort  Tag=PMCPort  Port=6  Side=Right
  wires:
  "PMU (PLL-Based, Positive-Sequence)1"/3 -> To Workspace5/1
  "PMU (PLL-Based, Positive-Sequence)1"/2 -> To Workspace4/1
  "PMU (PLL-Based, Positive-Sequence)1"/1 -> To Workspace3/1
  "PMU (PLL-Based, Positive-Sequence)2"/3 -> To Workspace6/1
  "PMU (PLL-Based, Positive-Sequence)2"/1 -> To Workspace1/1
  "PMU (PLL-Based, Positive-Sequence)2"/2 -> To Workspace2/1
  Three-Phase V-I Measurement25/1 -> "PMU (PLL-Based, Positive-Sequence)2"/1
  Three-Phase V-I Measurement1/1 -> "PMU (PLL-Based, Positive-Sequence)1"/1
  connections:
  Three-Phase V-I Measurement25/LConn1 -- Connection Port/RConn1 -- Three-Phase V-I Measurement1/LConn1
  Connection Port1/RConn1 -- Three-Phase V-I Measurement1/LConn2 -- Three-Phase V-I Measurement25/LConn2
  Connection Port2/RConn1 -- Three-Phase V-I Measurement25/LConn3 -- Three-Phase V-I Measurement1/LConn3
  Connection Port3/RConn1 -- Three-Phase V-I Measurement25/RConn1
  Three-Phase V-I Measurement25/RConn2 -- Connection Port4/RConn1
  Three-Phase V-I Measurement25/RConn3 -- Connection Port5/RConn1

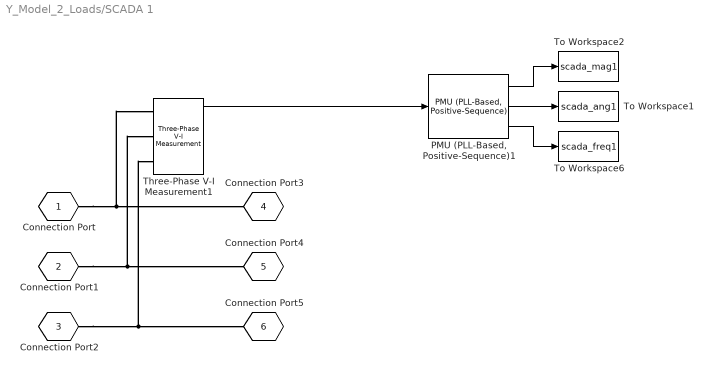
== system Y_Model_2_Loads/SCADA 1 ==
  "PMU (PLL-Based, Positive-Sequence)1" : powerlib_meascontrol/Measurements/PMU (PLL-Based, Positive-Sequence)  nominalFrequency=50  samplingRate=64  reportingFactor=1280
      settings: SourceProductName=Simscape Electrical  SourceProductBaseCode=PS
  Three-Phase V-I Measurement1 : powerlib/Measurements/Three-Phase V-I Measurement  VoltageMeasurement=phase-to-ground  SetLabelV=off  LabelV=Vabc  Vpu=off  VpuLL=off  CurrentMeasurement=no  SetLabelI=off  LabelI=Iabc  Ipu=off  Pbase=100e6  Vbase=500e3  OutputType=Complex  PhasorSimulation=off  PSBequivalent=0
      settings: SourceProductName=Simscape Electrical
  To Workspace1 : ToWorkspace  VariableName=scada_ang1  SampleTime=-1
  To Workspace2 : ToWorkspace  VariableName=scada_mag1  SampleTime=-1
  To Workspace6 : ToWorkspace  VariableName=scada_freq1  SampleTime=-1
  Connection Port : PMIOPort  Tag=PMCPort  Side=Left
  Connection Port1 : PMIOPort  Tag=PMCPort  Port=2  Side=Left
  Connection Port2 : PMIOPort  Tag=PMCPort  Port=3  Side=Left
  Connection Port3 : PMIOPort  Tag=PMCPort  Port=4  Side=Right
  Connection Port4 : PMIOPort  Tag=PMCPort  Port=5  Side=Right
  Connection Port5 : PMIOPort  Tag=PMCPort  Port=6  Side=Right
  wires:
  Three-Phase V-I Measurement1/1 -> "PMU (PLL-Based, Positive-Sequence)1"/1
  "PMU (PLL-Based, Positive-Sequence)1"/1 -> To Workspace2/1
  "PMU (PLL-Based, Positive-Sequence)1"/2 -> To Workspace1/1
  "PMU (PLL-Based, Positive-Sequence)1"/3 -> To Workspace6/1
  connections:
  Connection Port/RConn1 -- Connection Port3/RConn1 -- Three-Phase V-I Measurement1/LConn1
  Connection Port1/RConn1 -- Connection Port4/RConn1 -- Three-Phase V-I Measurement1/LConn2
  Connection Port2/RConn1 -- Three-Phase V-I Measurement1/LConn3 -- Connection Port5/RConn1

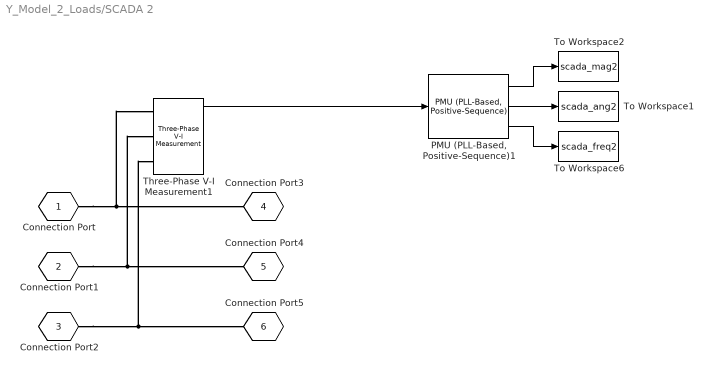
== system Y_Model_2_Loads/SCADA 2 ==
  "PMU (PLL-Based, Positive-Sequence)1" : powerlib_meascontrol/Measurements/PMU (PLL-Based, Positive-Sequence)  nominalFrequency=50  samplingRate=64  reportingFactor=1280
      settings: SourceProductName=Simscape Electrical  SourceProductBaseCode=PS
  Three-Phase V-I Measurement1 : powerlib/Measurements/Three-Phase V-I Measurement  VoltageMeasurement=phase-to-ground  SetLabelV=off  LabelV=Vabc  Vpu=off  VpuLL=off  CurrentMeasurement=no  SetLabelI=off  LabelI=Iabc  Ipu=off  Pbase=100e6  Vbase=500e3  OutputType=Complex  PhasorSimulation=off  PSBequivalent=0
      settings: SourceProductName=Simscape Electrical
  To Workspace1 : ToWorkspace  VariableName=scada_ang2  SampleTime=-1
  To Workspace2 : ToWorkspace  VariableName=scada_mag2  SampleTime=-1
  To Workspace6 : ToWorkspace  VariableName=scada_freq2  SampleTime=-1
  Connection Port : PMIOPort  Tag=PMCPort  Side=Left
  Connection Port1 : PMIOPort  Tag=PMCPort  Port=2  Side=Left
  Connection Port2 : PMIOPort  Tag=PMCPort  Port=3  Side=Left
  Connection Port3 : PMIOPort  Tag=PMCPort  Port=4  Side=Right
  Connection Port4 : PMIOPort  Tag=PMCPort  Port=5  Side=Right
  Connection Port5 : PMIOPort  Tag=PMCPort  Port=6  Side=Right
  wires:
  Three-Phase V-I Measurement1/1 -> "PMU (PLL-Based, Positive-Sequence)1"/1
  "PMU (PLL-Based, Positive-Sequence)1"/1 -> To Workspace2/1
  "PMU (PLL-Based, Positive-Sequence)1"/2 -> To Workspace1/1
  "PMU (PLL-Based, Positive-Sequence)1"/3 -> To Workspace6/1
  connections:
  Connection Port/RConn1 -- Connection Port3/RConn1 -- Three-Phase V-I Measurement1/LConn1
  Connection Port1/RConn1 -- Connection Port4/RConn1 -- Three-Phase V-I Measurement1/LConn2
  Connection Port2/RConn1 -- Three-Phase V-I Measurement1/LConn3 -- Connection Port5/RConn1

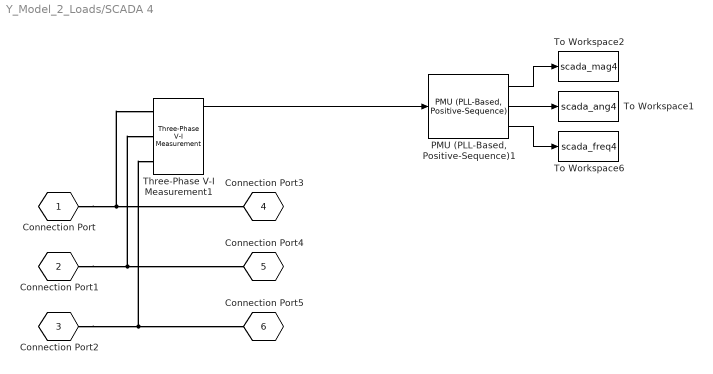
== system Y_Model_2_Loads/SCADA 4 ==
  "PMU (PLL-Based, Positive-Sequence)1" : powerlib_meascontrol/Measurements/PMU (PLL-Based, Positive-Sequence)  nominalFrequency=50  samplingRate=64  reportingFactor=1280
      settings: SourceProductName=Simscape Electrical  SourceProductBaseCode=PS
  Three-Phase V-I Measurement1 : powerlib/Measurements/Three-Phase V-I Measurement  VoltageMeasurement=phase-to-ground  SetLabelV=off  LabelV=Vabc  Vpu=off  VpuLL=off  CurrentMeasurement=no  SetLabelI=off  LabelI=Iabc  Ipu=off  Pbase=100e6  Vbase=500e3  OutputType=Complex  PhasorSimulation=off  PSBequivalent=0
      settings: SourceProductName=Simscape Electrical
  To Workspace1 : ToWorkspace  VariableName=scada_ang4  SampleTime=-1
  To Workspace2 : ToWorkspace  VariableName=scada_mag4  SampleTime=-1
  To Workspace6 : ToWorkspace  VariableName=scada_freq4  SampleTime=-1
  Connection Port : PMIOPort  Tag=PMCPort  Side=Left
  Connection Port1 : PMIOPort  Tag=PMCPort  Port=2  Side=Left
  Connection Port2 : PMIOPort  Tag=PMCPort  Port=3  Side=Left
  Connection Port3 : PMIOPort  Tag=PMCPort  Port=4  Side=Right
  Connection Port4 : PMIOPort  Tag=PMCPort  Port=5  Side=Right
  Connection Port5 : PMIOPort  Tag=PMCPort  Port=6  Side=Right
  wires:
  Three-Phase V-I Measurement1/1 -> "PMU (PLL-Based, Positive-Sequence)1"/1
  "PMU (PLL-Based, Positive-Sequence)1"/1 -> To Workspace2/1
  "PMU (PLL-Based, Positive-Sequence)1"/2 -> To Workspace1/1
  "PMU (PLL-Based, Positive-Sequence)1"/3 -> To Workspace6/1
  connections:
  Connection Port/RConn1 -- Connection Port3/RConn1 -- Three-Phase V-I Measurement1/LConn1
  Connection Port1/RConn1 -- Connection Port4/RConn1 -- Three-Phase V-I Measurement1/LConn2
  Connection Port2/RConn1 -- Three-Phase V-I Measurement1/LConn3 -- Connection Port5/RConn1
